simulink model "RegLab1_3mod"  (R2024a)
settings: Solver=VariableStepAuto  StartTime=0.0  StopTime=4200  RelTol=1e-3
model workspace (MAT data in the model file):
  param_K1 = 0.025
  param_K2 = 1.73913043478
  param_tau = 900
values from neighbouring files (symbols this model uses):
  u_aus = -0.02    [RegLab1_3.m]
  u_ein = 0.02    [RegLab1_3.m]
settings Model: Creator=maile  LastModifiedBy=maile

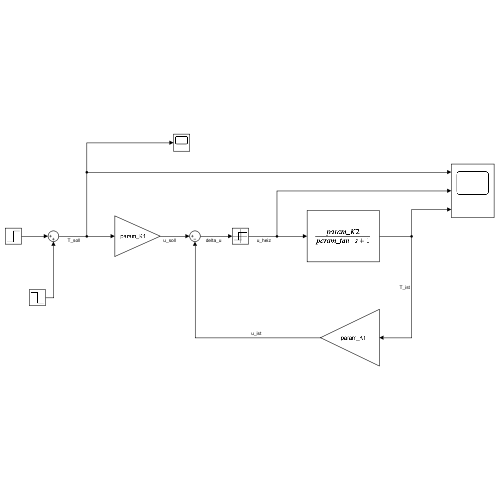
[thumbnail: Simulink's stored preview of the top-level diagram]
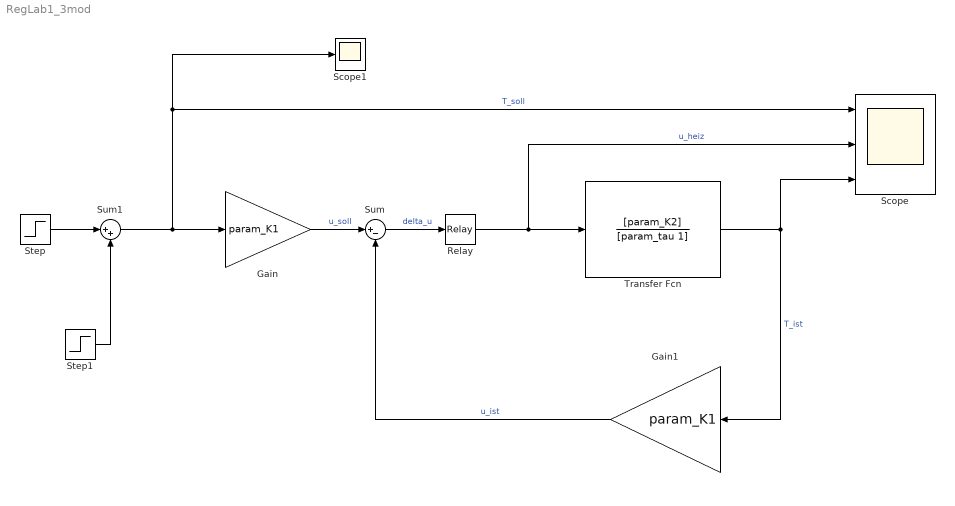
== system RegLab1_3mod ==
  Gain : Gain  Gain=param_K1
  Gain1 : Gain  Gain=param_K1
  Relay : Relay  OnSwitchValue=u_ein  OffSwitchValue=u_aus  OnOutputValue=230
  Scope : Scope  NumInputPorts=3
  Scope1 : Scope
  Step : Step  Time=0  After=160  SampleTime=0
  Step1 : Step  Time=1800  After=-160  SampleTime=0
  Sum : Sum  Inputs=|+-
  Sum1 : Sum  Inputs=|++
  Transfer Fcn : TransferFcn  Numerator=[param_K2]  Denominator=[param_tau 1]
  wires:
  Step/1 -> Sum1/1
  Sum1/1 -> Scope1/1, Scope/1, Gain/1  "T_soll"
  Relay/1 -> Scope/2, Transfer Fcn/1  "u_heiz"
  Transfer Fcn/1 -> Scope/3, Gain1/1  "T_ist"
  Gain/1 -> Sum/1  "u_soll"
  Sum/1 -> Relay/1  "delta_u"
  Gain1/1 -> Sum/2  "u_ist"
  Step1/1 -> Sum1/2
